simulink model "Nonlinear_TestHarness"  (R2024b)
settings: Solver=VariableStepAuto  StartTime=0.0  StopTime=10  RelTol=1e-3
undefined symbols (not defined in the file or in its folder): AC, Aero, ft, in, initVb, s
libraries: aerolibconvert2 x6, aerolibasang x3, simulink_extras x3, aerolibtransform2 x2, shared6dof x1, aerolibadyn x1, vrlib x1
settings Model: Creator=Jay  LastModifiedBy=jaycastruita

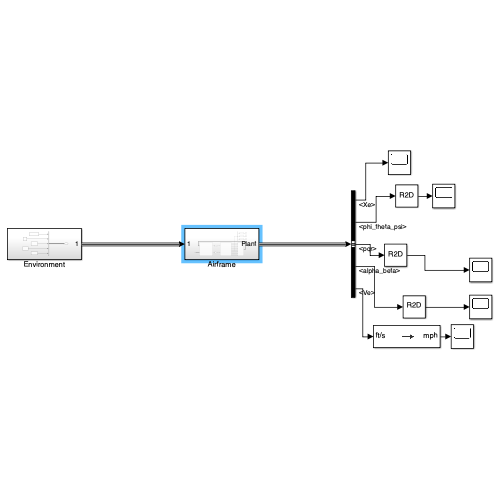
[thumbnail: Simulink's stored preview of the top-level diagram]
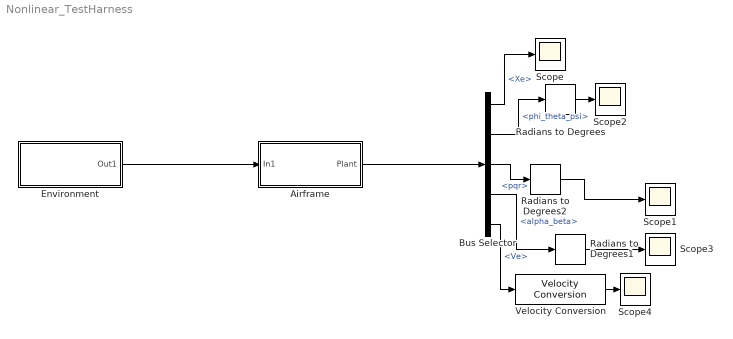
== system Nonlinear_TestHarness ==
  Airframe : Subsystem
  Bus Selector : BusSelector  OutputSignals=Xe,phi_theta_psi,pqr,alpha_beta,Ve
  Environment : Subsystem
  Radians to Degrees : simulink_extras/Transformations/Radians to Degrees
  Radians to Degrees1 : simulink_extras/Transformations/Radians to Degrees
  Radians to Degrees2 : simulink_extras/Transformations/Radians to Degrees
  Scope{,1..4} (5 alike) : Scope
  Velocity Conversion : aerolibconvert2/Velocity Conversion  IU=ft/s  OU=mph
  wires:
  Environment/1(Out1) -> Airframe/1(In1)
  Airframe/1(Plant) -> Bus Selector/1
  Bus Selector/1 -> Scope/1  "<Xe>"
  Bus Selector/3 -> Radians to Degrees2/1  "<pqr>"
  Bus Selector/2 -> Radians to Degrees/1  "<phi_theta_psi>"
  Radians to Degrees/1 -> Scope2/1
  Bus Selector/4 -> Radians to Degrees1/1  "<alpha_beta>"
  Radians to Degrees1/1 -> Scope3/1
  Radians to Degrees2/1 -> Scope1/1
  Bus Selector/5 -> Velocity Conversion/1  "<Ve>"
  Velocity Conversion/1 -> Scope4/1

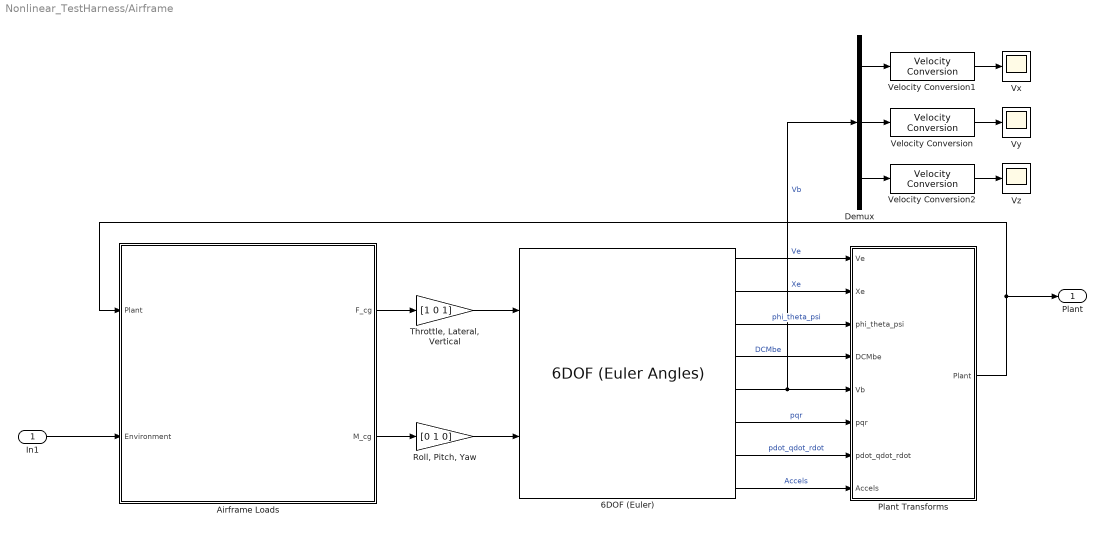
== system Nonlinear_TestHarness/Airframe ==
  In1 : Inport
  6DOF (Euler) : shared6dof/6DOF (Euler Angles)  units=English (Velocity in ft/s)  mtype=Fixed  rep=Euler Angles  xme_0=[0 0 0]  Vm_0=initVb  eul_0=[0 0 0]  pm_0=[0 0 0]  mass_0=AC.mass  mass_e=0.5  mass_f=2.0  inertia=AC.Inertia  inertia_e=eye(3)  inertia_f=2*eye(3)  k_quat=1.0  vre_flag=on  abi_flag=off  aMode=0  xme_statename=''  Vm_statename=''  eul_statename=''  quat_statename=''  pm_statename=''  mass_statename=''
      settings: LibrarySourceBlock=aerolib6dof2/6DOF (Quaternion)
  Airframe Loads : Subsystem
  Demux : Demux  Outputs=3
  Plant Transforms : Subsystem
  "Roll, Pitch, Yaw" : Gain  Gain=[0 1 0]
  "Throttle, Lateral, Vertical" : Gain  Gain=[1 0 1]
  Velocity Conversion : aerolibconvert2/Velocity Conversion  IU=ft/s  OU=mph
  Velocity Conversion1 : aerolibconvert2/Velocity Conversion  IU=ft/s  OU=mph
  Velocity Conversion2 : aerolibconvert2/Velocity Conversion  IU=ft/s  OU=mph
  Vx : Scope
  Vy : Scope
  Vz : Scope
  Plant : Outport
  wires:
  In1/1 -> Airframe Loads/2(Environment)
  Airframe Loads/1(F_cg) -> "Throttle, Lateral, Vertical"/1
  6DOF (Euler)/1 -> Plant Transforms/1(Ve)  "Ve"
  6DOF (Euler)/2 -> Plant Transforms/2(Xe)  "Xe"
  6DOF (Euler)/3 -> Plant Transforms/3(phi_theta_psi)  "phi_theta_psi"
  6DOF (Euler)/5 -> Demux/1, Plant Transforms/5(Vb)  "Vb"
  6DOF (Euler)/4 -> Plant Transforms/4(DCMbe)  "DCMbe"
  6DOF (Euler)/6 -> Plant Transforms/6(pqr)  "pqr"
  6DOF (Euler)/7 -> Plant Transforms/7(pdot_qdot_rdot)  "pdot_qdot_rdot"
  6DOF (Euler)/8 -> Plant Transforms/8(Accels)  "Accels"
  Plant Transforms/1(Plant) -> Airframe Loads/1(Plant), Plant/1
  Airframe Loads/2(M_cg) -> "Roll, Pitch, Yaw"/1
  "Roll, Pitch, Yaw"/1 -> 6DOF (Euler)/2
  "Throttle, Lateral, Vertical"/1 -> 6DOF (Euler)/1
  Demux/1 -> Velocity Conversion1/1
  Demux/2 -> Velocity Conversion/1
  Demux/3 -> Velocity Conversion2/1
  Velocity Conversion/1 -> Vy/1
  Velocity Conversion1/1 -> Vx/1
  Velocity Conversion2/1 -> Vz/1

== system Nonlinear_TestHarness/Environment ==
  Air Density : Constant  Value=0.002377
  Bus Creator : BusCreator  Inputs=5
  Gravity : Constant  Value=[0 0 32.2]
  Speed of Sound : Constant  Value=1100
  Wind Angular Rates : Constant  Value=[0 0 0]
  Wind Velocity : Constant  Value=[0 0 0]
  Out1 : Outport
  wires:
  Wind Velocity/1 -> Bus Creator/4  "WindVelocity"
  Speed of Sound/1 -> Bus Creator/2  "a"
  Air Density/1 -> Bus Creator/3  "rho"
  Bus Creator/1 -> Out1/1  "Environment"
  Wind Angular Rates/1 -> Bus Creator/5  "WindAngularRates"
  Gravity/1 -> Bus Creator/1  "Ag"

== system Nonlinear_TestHarness/Airframe/Airframe Loads ==
  Plant : Inport
  In Bus Element : Inport  Port=2  PortName=Environment
  Add : Sum
  Aerodynamic Loads : Subsystem
  Gravity Force : Subsystem
  F_cg : Outport
  M_cg : Outport  Port=2
  wires:
  Plant/1 -> Gravity Force/1(Plant), Aerodynamic Loads/2(plant)
  In Bus Element/1 -> Gravity Force/2(Environment), Aerodynamic Loads/1(EnvData)
  Aerodynamic Loads/1(Fb) -> Add/1
  Add/1 -> F_cg/1
  Gravity Force/1(Fg_b) -> Add/2
  Aerodynamic Loads/2(Mb) -> M_cg/1

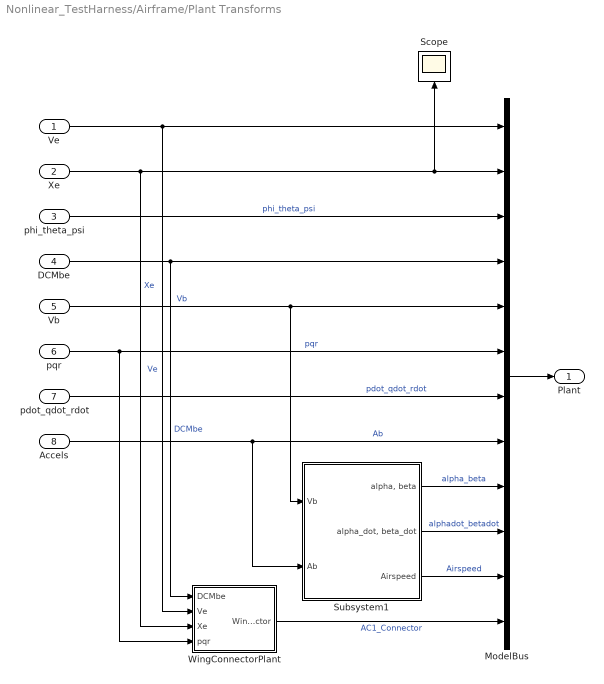
== system Nonlinear_TestHarness/Airframe/Plant Transforms ==
  Ve : Inport
  Xe : Inport  Port=2
  phi_theta_psi : Inport  Port=3
  DCMbe : Inport  Port=4
  Vb : Inport  Port=5
  pqr : Inport  Port=6
  pdot_qdot_rdot : Inport  Port=7
  Accels : Inport  Port=8
  ModelBus : BusCreator  Inputs=12
  Scope : Scope
  Subsystem1 : Subsystem
  WingConnectorPlant : Subsystem
  Plant : Outport
  wires:
  Ve/1 -> WingConnectorPlant/2(Ve), ModelBus/1  "Ve"
  ModelBus/1 -> Plant/1
  DCMbe/1 -> ModelBus/4, WingConnectorPlant/1(DCMbe)  "DCMbe"
  pqr/1 -> WingConnectorPlant/4(pqr), ModelBus/6  "pqr"
  pdot_qdot_rdot/1 -> ModelBus/7  "pdot_qdot_rdot"
  Subsystem1/2("alpha_dot, beta_dot") -> ModelBus/10  "alphadot_betadot"
  WingConnectorPlant/1(WingConnector) -> ModelBus/12  "AC1_Connector"
  Xe/1 -> WingConnectorPlant/3(Xe), ModelBus/2, Scope/1  "Xe"
  Subsystem1/1("alpha, beta") -> ModelBus/9  "alpha_beta"
  phi_theta_psi/1 -> ModelBus/3  "phi_theta_psi"
  Accels/1 -> Subsystem1/2(Ab), ModelBus/8  "Ab"
  Vb/1 -> Subsystem1/1(Vb), ModelBus/5  "Vb"
  Subsystem1/3(Airspeed) -> ModelBus/11  "Airspeed"

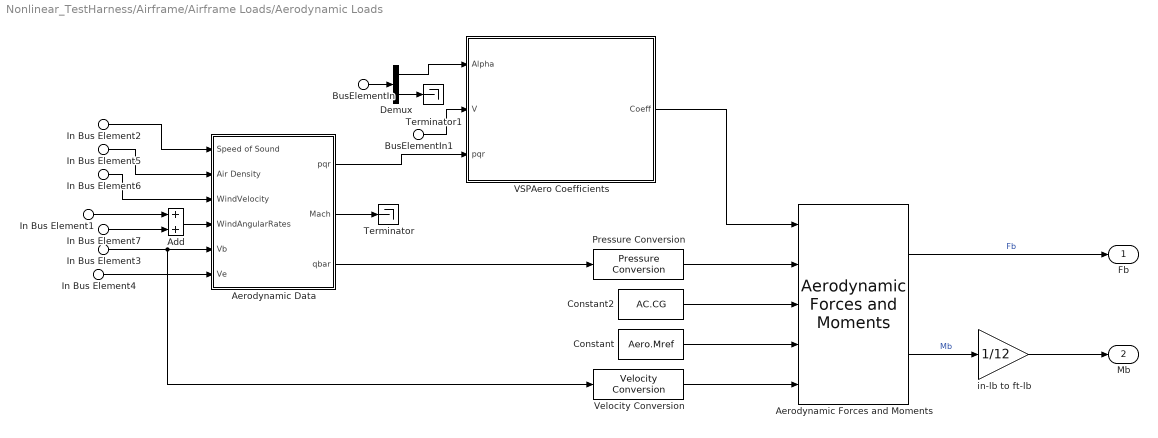
== system Nonlinear_TestHarness/Airframe/Airframe Loads/Aerodynamic Loads ==
  In Bus Element6 : Inport  PortName=EnvData  Element=WindVelocity
  In Bus Element7 : Inport  PortName=EnvData  Element=WindAngularRates
  In Bus Element2 : Inport  PortName=EnvData  Element=a
  In Bus Element5 : Inport  PortName=EnvData  Element=rho
  In Bus Element3 : Inport  Port=2  PortName=plant  Element=Vb
  In Bus Element4 : Inport  Port=2  PortName=plant  Element=Ve
  In Bus Element1 : Inport  Port=2  PortName=plant  Element=pqr
  BusElementIn : Inport  Port=2  PortName=plant  Element=alpha_beta
  BusElementIn1 : Inport  Port=2  PortName=plant  Element=Airspeed
  Add : Sum
  Aerodynamic Forces and Moments : aerolibadyn/Aerodynamic Forces and Moments   inputAxes=Wind  outputForceAxes=Body  outputMomentAxes=Body  S=Aero.Sref  b=Aero.bref  cbar=Aero.Cref
  Aerodynamic Data : Subsystem
  Constant : Constant  Value=Aero.Mref
  Constant2 : Constant  Value=AC.CG
  Demux : Demux  Outputs=2
  Pressure Conversion : aerolibconvert2/Pressure Conversion  IU=psf  OU=psi
  Terminator : Terminator
  Terminator1 : Terminator
  VSPAero Coefficients : Subsystem
  Velocity Conversion : aerolibconvert2/Velocity Conversion  IU=ft/s  OU=in/s
  in-lb to ft-lb : Gain  Gain=1/12
  Fb : Outport  VectorParamsAs1DForOutWhenUnconnected=off
  Mb : Outport  Port=2  VectorParamsAs1DForOutWhenUnconnected=off
  wires:
  In Bus Element6/1 -> Aerodynamic Data/3(WindVelocity)
  Aerodynamic Data/1("pqr ") -> VSPAero Coefficients/3(pqr)
  Aerodynamic Forces and Moments/2 -> in-lb to ft-lb/1  "Mb"
  VSPAero Coefficients/1(Coeff) -> Aerodynamic Forces and Moments/1
  In Bus Element7/1 -> Add/2
  Constant/1 -> Aerodynamic Forces and Moments/4
  In Bus Element5/1 -> Aerodynamic Data/2(Air Density)
  In Bus Element2/1 -> Aerodynamic Data/1(Speed of Sound)
  Add/1 -> Aerodynamic Data/4(WindAngularRates)
  In Bus Element4/1 -> Aerodynamic Data/6(Ve)
  Aerodynamic Forces and Moments/1 -> Fb/1  "Fb"
  In Bus Element1/1 -> Add/1
  BusElementIn/1 -> Demux/1
  Demux/1 -> VSPAero Coefficients/1(Alpha)
  In Bus Element3/1 -> Velocity Conversion/1, Aerodynamic Data/5(Vb)
  Aerodynamic Data/3(qbar) -> Pressure Conversion/1
  Constant2/1 -> Aerodynamic Forces and Moments/3
  Pressure Conversion/1 -> Aerodynamic Forces and Moments/2
  Velocity Conversion/1 -> Aerodynamic Forces and Moments/5
  in-lb to ft-lb/1 -> Mb/1
  Aerodynamic Data/2(Mach) -> Terminator/1
  Demux/2 -> Terminator1/1
  BusElementIn1/1 -> VSPAero Coefficients/2(V)

== system Nonlinear_TestHarness/Airframe/Airframe Loads/Gravity Force ==
  Plant : Inport
  Bus Element In2 : Inport  Port=2  PortName=Environment
  Acc to Force : Gain  Gain=AC.mass  OutDataTypeStr=Inherit: Same as input  ParamDataTypeStr=Inherit: Same as input
  Bus Selector : BusSelector  OutputSignals=DCMbe
  Bus Selector1 : BusSelector  OutputSignals=Ag
  Fg_body : Product  Multiplication=Matrix(*)
  Fg_b : Outport
  wires:
  Bus Selector/1 -> Fg_body/1  "<DCMbe>"
  Acc to Force/1 -> Fg_body/2
  Plant/1 -> Bus Selector/1
  Bus Element In2/1 -> Bus Selector1/1
  Bus Selector1/1 -> Acc to Force/1  "<Ag>"
  Fg_body/1 -> Fg_b/1

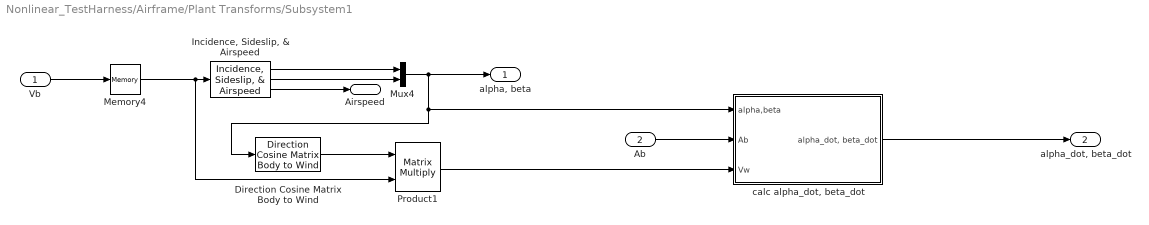
== system Nonlinear_TestHarness/Airframe/Plant Transforms/Subsystem1 ==
  Vb : Inport
  Ab : Inport  Port=2
  Direction Cosine Matrix Body to Wind : aerolibtransform2/Direction Cosine Matrix Body to Wind
  "Incidence, Sideslip, & Airspeed" : aerolibasang/Incidence, Sideslip, & Airspeed
  Memory4 : Memory  InitialCondition=initVb
  Mux4 : Mux  Inputs=2
  Product1 : Product  Multiplication=Matrix(*)  InputSameDT=on  SaturateOnIntegerOverflow=on  OutDataTypeStr=Inherit: Same as first input
  "calc alpha_dot, beta_dot" : Subsystem
  "alpha, beta" : Outport  Unit=rad  VectorParamsAs1DForOutWhenUnconnected=off
  "alpha_dot, beta_dot" : Outport  Port=2  Unit=rad/s  VectorParamsAs1DForOutWhenUnconnected=off
  Airspeed : Outport  Port=3
  wires:
  "Incidence, Sideslip, & Airspeed"/2 -> Mux4/2
  Mux4/1 -> "alpha, beta"/1, Direction Cosine Matrix Body to Wind/1, "calc alpha_dot, beta_dot"/1(alpha,beta)
  Direction Cosine Matrix Body to Wind/1 -> Product1/1
  "Incidence, Sideslip, & Airspeed"/1 -> Mux4/1
  Memory4/1 -> Product1/2, "Incidence, Sideslip, & Airspeed"/1
  Product1/1 -> "calc alpha_dot, beta_dot"/3(Vw)
  Ab/1 -> "calc alpha_dot, beta_dot"/2(Ab)
  "Incidence, Sideslip, & Airspeed"/3 -> Airspeed/1
  "calc alpha_dot, beta_dot"/1("alpha_dot, beta_dot") -> "alpha_dot, beta_dot"/1
  Vb/1 -> Memory4/1

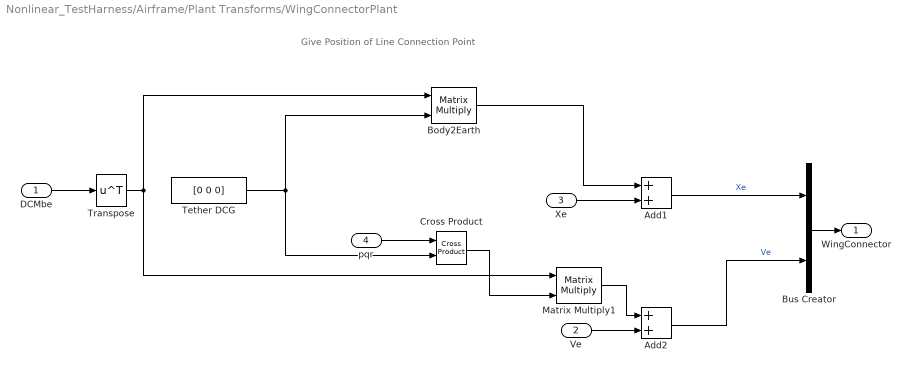
== system Nonlinear_TestHarness/Airframe/Plant Transforms/WingConnectorPlant ==
  note: Give Position of Line Connection Point
  DCMbe : Inport
  Ve : Inport  Port=2
  Xe : Inport  Port=3
  pqr : Inport  Port=4
  Add1 : Sum
  Add2 : Sum
  Body2Earth : Product  Multiplication=Matrix(*)
  Bus Creator : BusCreator  Inputs=2
  Cross Product : vrlib/Utilities/Cross Product
  Matrix Multiply1 : Product  Multiplication=Matrix(*)
  Tether DCG : Constant  Value=[0 0 0]
  Transpose : Math  Operator=transpose
  WingConnector : Outport
  wires:
  Bus Creator/1 -> WingConnector/1
  Transpose/1 -> Body2Earth/1, Matrix Multiply1/1
  Body2Earth/1 -> Add1/1
  Add2/1 -> Bus Creator/2  "Ve"
  Xe/1 -> Add1/2
  Matrix Multiply1/1 -> Add2/1
  Tether DCG/1 -> Cross Product/2, Body2Earth/2
  pqr/1 -> Cross Product/1
  Cross Product/1 -> Matrix Multiply1/2
  Add1/1 -> Bus Creator/1  "Xe"
  DCMbe/1 -> Transpose/1
  Ve/1 -> Add2/2

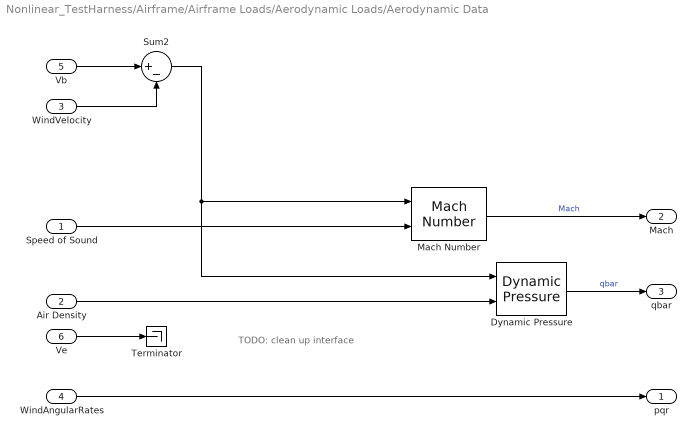
== system Nonlinear_TestHarness/Airframe/Airframe Loads/Aerodynamic Loads/Aerodynamic Data ==
  note: TODO: clean up interface
  Speed of Sound : Inport
  Air Density : Inport  Port=2
  WindVelocity : Inport  Port=3  PortDimensions=3
  WindAngularRates : Inport  Port=4  PortDimensions=3
  Vb : Inport  Port=5  PortDimensions=3
  Ve : Inport  Port=6  PortDimensions=3
  Dynamic Pressure : aerolibasang/Dynamic Pressure
  Mach Number : aerolibasang/Mach Number
  Sum2 : Sum  Inputs=|+-  InputSameDT=on  SaturateOnIntegerOverflow=on  OutDataTypeStr=Inherit: Same as first input
  Terminator : Terminator
  "pqr " : Outport  VectorParamsAs1DForOutWhenUnconnected=off
  Mach : Outport  Port=2  VectorParamsAs1DForOutWhenUnconnected=off
  qbar : Outport  Port=3  VectorParamsAs1DForOutWhenUnconnected=off
  wires:
  Dynamic Pressure/1 -> qbar/1  "qbar"
  Sum2/1 -> Mach Number/1, Dynamic Pressure/1
  Ve/1 -> Terminator/1
  Mach Number/1 -> Mach/1  "Mach"
  WindVelocity/1 -> Sum2/2
  Air Density/1 -> Dynamic Pressure/2
  WindAngularRates/1 -> "pqr "/1
  Speed of Sound/1 -> Mach Number/2
  Vb/1 -> Sum2/1

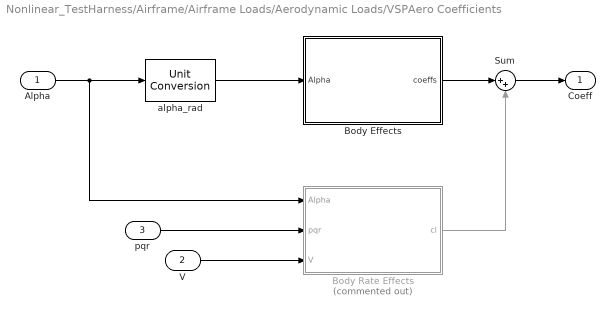
== system Nonlinear_TestHarness/Airframe/Airframe Loads/Aerodynamic Loads/VSPAero Coefficients ==
  Alpha : Inport  Unit=rad
  V : Inport  Port=2
  pqr : Inport  Port=3
  Body Effects : Subsystem
  Body Rate Effects : Subsystem  Commented=on
  Sum : Sum  Inputs=|++
  alpha_rad : UnitConversion
  Coeff : Outport  VectorParamsAs1DForOutWhenUnconnected=off
  wires:
  alpha_rad/1 -> Body Effects/1(Alpha)
  Alpha/1 -> Body Rate Effects/1(Alpha), alpha_rad/1
  Body Effects/1(coeffs) -> Sum/1
  Sum/1 -> Coeff/1
  pqr/1 -> Body Rate Effects/2(pqr)
  V/1 -> Body Rate Effects/3(V)
  Body Rate Effects/1(cl) -> Sum/2

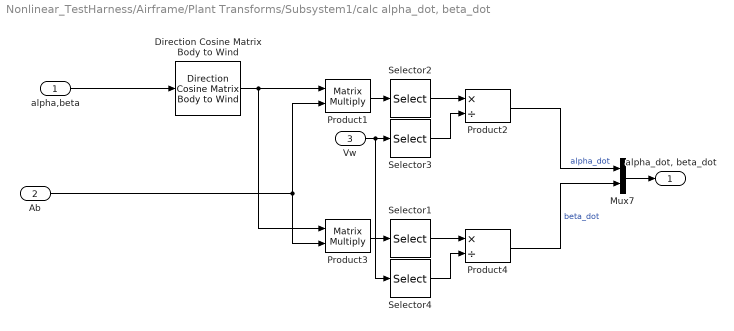
== system Nonlinear_TestHarness/Airframe/Plant Transforms/Subsystem1/calc alpha_dot, beta_dot ==
  alpha,beta : Inport
  Ab : Inport  Port=2
  Vw : Inport  Port=3
  Direction Cosine Matrix Body to Wind : aerolibtransform2/Direction Cosine Matrix Body to Wind
  Mux7 : Mux  Inputs=2
  Product1 : Product  Multiplication=Matrix(*)  InputSameDT=on  SaturateOnIntegerOverflow=on  OutDataTypeStr=Inherit: Same as first input
  Product2 : Product  Inputs=*/  InputSameDT=on  SaturateOnIntegerOverflow=on  OutDataTypeStr=Inherit: Same as first input
  Product3 : Product  Multiplication=Matrix(*)  InputSameDT=on  SaturateOnIntegerOverflow=on  OutDataTypeStr=Inherit: Same as first input
  Product4 : Product  Inputs=*/  InputSameDT=on  SaturateOnIntegerOverflow=on  OutDataTypeStr=Inherit: Same as first input
  Selector1 : Selector  IndexMode=Zero-based  InputPortWidth=3  IndexOptions=Index vector (dialog)  Indices=1  OutputSizes=1
  Selector2 : Selector  IndexMode=Zero-based  InputPortWidth=3  IndexOptions=Index vector (dialog)  Indices=2  OutputSizes=1
  Selector3 : Selector  IndexMode=Zero-based  InputPortWidth=3  IndexOptions=Index vector (dialog)  Indices=0  OutputSizes=1
  Selector4 : Selector  IndexMode=Zero-based  InputPortWidth=3  IndexOptions=Index vector (dialog)  Indices=0  OutputSizes=1
  "alpha_dot, beta_dot" : Outport  VectorParamsAs1DForOutWhenUnconnected=off
  wires:
  Product1/1 -> Selector2/1
  Selector2/1 -> Product2/1
  Selector3/1 -> Product2/2
  alpha,beta/1 -> Direction Cosine Matrix Body to Wind/1
  Product2/1 -> Mux7/1  "alpha_dot"
  Ab/1 -> Product1/2, Product3/2
  Vw/1 -> Selector4/1, Selector3/1
  Product4/1 -> Mux7/2  "beta_dot"
  Direction Cosine Matrix Body to Wind/1 -> Product3/1, Product1/1
  Selector1/1 -> Product4/1
  Selector4/1 -> Product4/2
  Product3/1 -> Selector1/1
  Mux7/1 -> "alpha_dot, beta_dot"/1

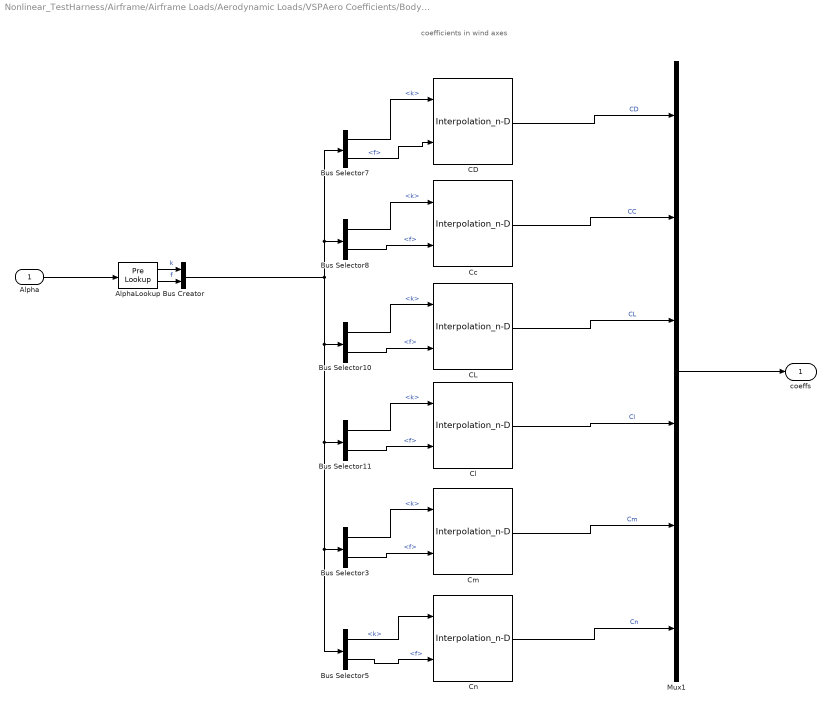
== system Nonlinear_TestHarness/Airframe/Airframe Loads/Aerodynamic Loads/VSPAero Coefficients/Body Effects ==
  note: coefficients in wind axes
  Alpha : Inport  Unit=deg
  AlphaLookup : PreLookup  BreakpointsData=Aero.alpha_vec  BeginIndexSearchUsingPreviousIndexResult=on  ExtrapMethod=Linear
  Bus Creator : BusCreator  Inputs=2
  Bus Selector{3,5,7..8,10..11} (6 alike) : BusSelector  OutputSignals=k,f
  CD : Interpolation_n-D  NumberOfTableDimensions=1  Table=Aero.CD  DiagnosticForOutOfRangeInput=Warning  RemoveProtectionIndex=on  SaturateOnIntegerOverflow=on
      settings: InputPortMap=u0,u1
  CL : Interpolation_n-D  NumberOfTableDimensions=1  Table=Aero.CL  ExtrapMethod=Clip  DiagnosticForOutOfRangeInput=Warning  RemoveProtectionIndex=on  SaturateOnIntegerOverflow=on
      settings: InputPortMap=u0,u1
  Cc : Interpolation_n-D  NumberOfTableDimensions=1  Table=Aero.Cc  RemoveProtectionIndex=on  SaturateOnIntegerOverflow=on
      settings: InputPortMap=u0,u1
  Cl : Interpolation_n-D  NumberOfTableDimensions=1  Table=Aero.Cl  RemoveProtectionIndex=on  SaturateOnIntegerOverflow=on
      settings: InputPortMap=u0,u1
  Cm : Interpolation_n-D  NumberOfTableDimensions=1  Table=Aero.Cm  ExtrapMethod=Clip  DiagnosticForOutOfRangeInput=Warning  RemoveProtectionIndex=on  SaturateOnIntegerOverflow=on
      settings: InputPortMap=u0,u1
  Cn : Interpolation_n-D  NumberOfTableDimensions=1  Table=Aero.Cn  RemoveProtectionIndex=on  SaturateOnIntegerOverflow=on
      settings: InputPortMap=u0,u1
  Mux1 : Mux  Inputs=6
  coeffs : Outport  VectorParamsAs1DForOutWhenUnconnected=off
  wires:
  AlphaLookup/2 -> Bus Creator/2  "f"
  AlphaLookup/1 -> Bus Creator/1  "k"
  Mux1/1 -> coeffs/1
  Alpha/1 -> AlphaLookup/1
  Cm/1 -> Mux1/5  "Cm"
  Bus Selector11/1 -> Cl/1  "<k>"
  Bus Selector8/1 -> Cc/1  "<k>"
  Bus Selector5/1 -> Cn/1  "<k>"
  Bus Selector11/2 -> Cl/2  "<f>"
  Bus Selector5/2 -> Cn/2  "<f>"
  Bus Selector7/1 -> CD/1  "<k>"
  Bus Selector3/2 -> Cm/2  "<f>"
  Bus Selector8/2 -> Cc/2  "<f>"
  CL/1 -> Mux1/3  "CL"
  Bus Selector10/1 -> CL/1  "<k>"
  Bus Selector7/2 -> CD/2  "<f>"
  Bus Selector10/2 -> CL/2  "<f>"
  Cn/1 -> Mux1/6  "Cn"
  Bus Creator/1 -> Bus Selector8/1, Bus Selector7/1, Bus Selector3/1, Bus Selector5/1, Bus Selector11/1, Bus Selector10/1
  Cc/1 -> Mux1/2  "CC"
  Bus Selector3/1 -> Cm/1  "<k>"
  Cl/1 -> Mux1/4  "Cl"
  CD/1 -> Mux1/1  "CD"

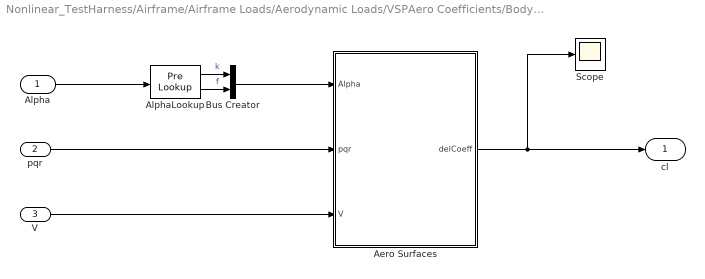
== system Nonlinear_TestHarness/Airframe/Airframe Loads/Aerodynamic Loads/VSPAero Coefficients/Body Rate Effects ==
  Alpha : Inport  Unit=deg
  pqr : Inport  Port=2
  V : Inport  Port=3
  Aero Surfaces : Subsystem
  AlphaLookup : PreLookup  BreakpointsData=Aero.alpha_vec  BeginIndexSearchUsingPreviousIndexResult=on  ExtrapMethod=Linear
  Bus Creator : BusCreator  Inputs=2
  Scope : Scope
  cl : Outport  VectorParamsAs1DForOutWhenUnconnected=off
  wires:
  V/1 -> Aero Surfaces/3(V)
  pqr/1 -> Aero Surfaces/2(pqr)
  AlphaLookup/2 -> Bus Creator/2  "f"
  AlphaLookup/1 -> Bus Creator/1  "k"
  Aero Surfaces/1(delCoeff) -> cl/1, Scope/1
  Alpha/1 -> AlphaLookup/1
  Bus Creator/1 -> Aero Surfaces/1(Alpha)

== system Nonlinear_TestHarness/Airframe/Airframe Loads/Aerodynamic Loads/VSPAero Coefficients/Body Rate Effects/Aero Surfaces ==
  note: C()_q
  Alpha : Inport
  pqr : Inport  Port=2
  V : Inport  Port=3
  Coefs Due to Pitch Rate : Subsystem
  Convert & Add : Subsystem
      settings: PortSchema="{\"entries\":[{\"content\":{\"sides\":[{\"content\":{\"connectorIds\":[\"In1\"]},\"type\":\"ConnectorPlacement.EquallySpacedRectSide\",\"uuid\":\"b8013de1-6e73-47c3-a52d-200a37bea422\"},{\"content\":{\"connectorIds\":[\"Out1\"],\"side\":\"RIGHT\"},\"type\":\"ConnectorPlacement.EquallySpacedRectSide\",\"uuid\":\"fcf5ea14-4050-433a-82d6-0b7656ed6099\"},{\"content\":{\"connectorIds\":[\"In2\",\"In3\"],\"side\":\"TOP\"},\"type\":\"ConnectorPlacement.EquallySpacedRectSide\",\"uuid\":\"1c09a769-a85c-46fb-a83d-04bd39ae92ac\"},{\"content\":{\"connectorIds\":[],\"side\":\"BOTTOM\"},\"type\":\"ConnectorPlacement.EquallySpacedRectSide\",\"uuid\":\"8f4a7c03-2c0e-435b-85d5-b3305cee738f\"}]},\"type\":\"ConnectorPlacement.EquallySpacedConnector\",\"uuid\":\"e7daaf90-0c94-4b5f-ae16-89aa994c358a\"}],\"packageUris\":[\"http://schema.mathworks.com/mf0/Connector/R2020b\"],\"version\":\"1.0\"}"
  delCoeff : Outport  VectorParamsAs1DForOutWhenUnconnected=off
  wires:
  Alpha/1 -> Coefs Due to Pitch Rate/1(Alpha)
  V/1 -> Convert & Add/3(V)
  Coefs Due to Pitch Rate/1(DampCoef) -> Convert & Add/1(DampCoef)
  pqr/1 -> Convert & Add/2(pqr)
  Convert & Add/1(delCoeff) -> delCoeff/1

== system Nonlinear_TestHarness/Airframe/Airframe Loads/Aerodynamic Loads/VSPAero Coefficients/Body Rate Effects/Aero Surfaces/Coefs Due to Pitch Rate ==
  note: "Flight Stability and Automatic Controls," by R. Nelson describes only 2 damping coefficients due to pitch rate. (Pg. 123): Z force, pitching moment
  Alpha : Inport
  Bus Selector11 : BusSelector  OutputSignals=k,f
  Cm_q : Interpolation_n-D  NumberOfTableDimensions=1  Table=Aero.Cm_q  ExtrapMethod=Clip  RemoveProtectionIndex=on  SaturateOnIntegerOverflow=on
      settings: InputPortMap=u0,u1
  Gain : Gain  Commented=through  Gain=0.1
  DampCoef : Outport
  wires:
  Bus Selector11/1 -> Cm_q/1  "<k>"
  Gain/1 -> DampCoef/1  "Cm_q"
  Bus Selector11/2 -> Cm_q/2  "<f>"
  Alpha/1 -> Bus Selector11/1
  Cm_q/1 -> Gain/1  "CMy"

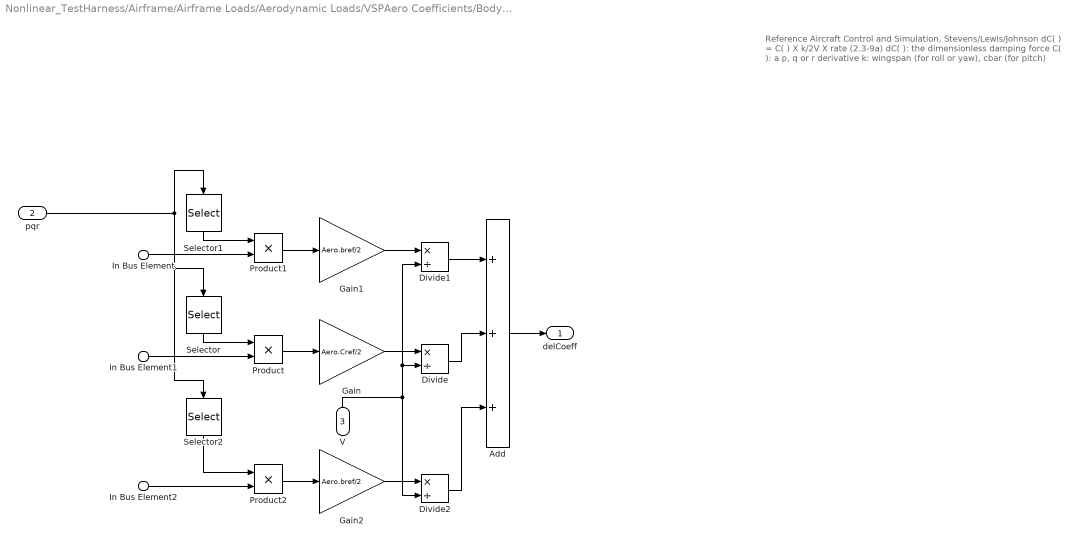
== system Nonlinear_TestHarness/Airframe/Airframe Loads/Aerodynamic Loads/VSPAero Coefficients/Body Rate Effects/Aero Surfaces/Convert & Add ==
  note: Reference Aircraft Control and Simulation, Stevens/Lewis/Johnson
      | dC( ) = C( ) X k/2V X rate    (2.3-9a)
      |
      | dC( ): the dimensionless damping force
      | C( ): a p, q or r derivative
      | k: wingspan (for roll or yaw), cbar (for pitch)
  In Bus Element : Inport  PortName=DampCoef  Element=C()_p
  In Bus Element1 : Inport  PortName=DampCoef  Element=C()_q
  In Bus Element2 : Inport  PortName=DampCoef  Element=C()_r
  pqr : Inport  Port=2
  V : Inport  Port=3
  Add : Sum  Inputs=+++
  Divide : Product  Inputs=*/
  Divide1 : Product  Inputs=*/
  Divide2 : Product  Inputs=*/
  Gain : Gain  Gain=Aero.Cref/2
  Gain1 : Gain  Gain=Aero.bref/2
  Gain2 : Gain  Gain=Aero.bref/2
  Product : Product
  Product1 : Product
  Product2 : Product
  Selector : Selector  InputPortWidth=3  IndexOptions=Index vector (dialog)  Indices=[ 2]  OutputSizes=1
  Selector1 : Selector  InputPortWidth=3  IndexOptions=Index vector (dialog)  Indices=[ 1]  OutputSizes=1
  Selector2 : Selector  InputPortWidth=3  IndexOptions=Index vector (dialog)  Indices=[ 3]  OutputSizes=1
  delCoeff : Outport
  wires:
  pqr/1 -> Selector1/1, Selector2/1, Selector/1
  Divide1/1 -> Add/1
  Selector/1 -> Product/1
  Selector1/1 -> Product1/1
  Gain1/1 -> Divide1/1
  Product1/1 -> Gain1/1
  Gain/1 -> Divide/1
  V/1 -> Divide2/2, Divide1/2, Divide/2
  Product/1 -> Gain/1
  In Bus Element2/1 -> Product2/2
  Divide/1 -> Add/2
  Divide2/1 -> Add/3
  Gain2/1 -> Divide2/1
  Product2/1 -> Gain2/1
  Add/1 -> delCoeff/1
  In Bus Element1/1 -> Product/2
  Selector2/1 -> Product2/1
  In Bus Element/1 -> Product1/2
